simulink model "System_Modell"  (R2018a)
settings: Solver=FixedStepAuto  StartTime=0.0  StopTime=inf  FixedStep=1/f  RelTol=1e-3
values from neighbouring files (symbols this model uses):
  f = 10000    [System_Init.m]
(part 2 of 8)

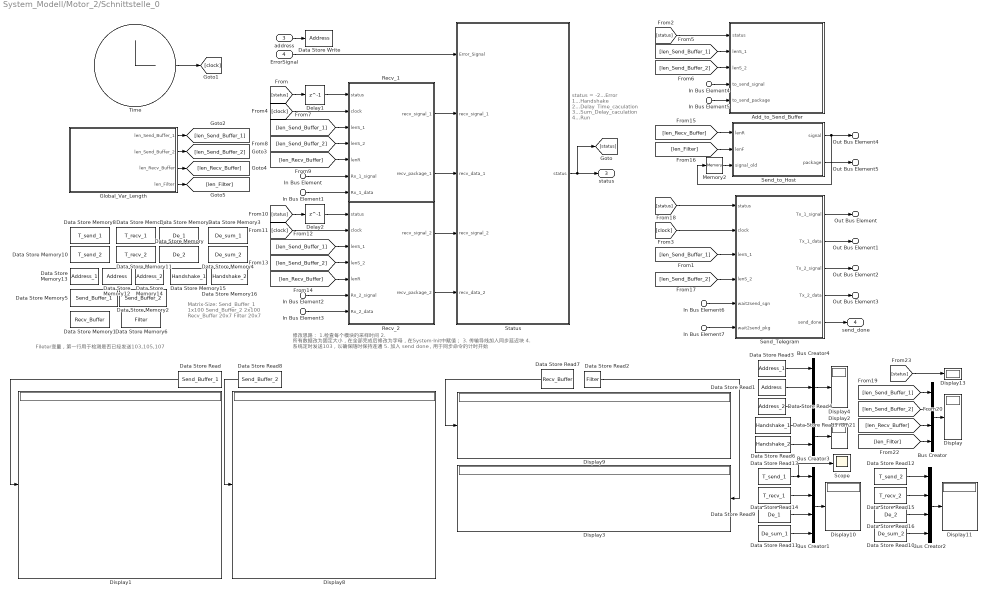
== system System_Modell/Motor_2/Schnittstelle_0 ==
  note: Fileter变量，第一行用于检测是否已经发送103,105,107
  note: 修改思路：
      | 1.检查每个模块的采样时间
      | 2. 所有数据改为固定大小，在全部完成后修改为字母，在System-Init中赋值；
      | 3. 传输导线加入同步延迟块
      | 4. 系统定时发送103，以确保随时保持连通
      | 5. 加入 send done，用于同步命令的计时开始
  note: status =
      | -2...Error
      |  1...Handshake
      |  2...Delay_Time_caculation
      |  3...Sum_Delay_caculation
      |  4...Run
  note: Matrix-Size:
      | Send_Buffer_1	1x100
      | Send_Buffer_2	2x100
      | Recv_Buffer		20x7
      | Filter			20x7
  In Bus Element : Inport  PortName=Rx_1  Element=signal
  In Bus Element1 : Inport  PortName=Rx_1  Element=data
  In Bus Element2 : Inport  Port=2  PortName=Rx_2  Element=signal
  In Bus Element3 : Inport  Port=2  PortName=Rx_2  Element=data
  address : Inport  Port=3
  ErrorSignal : Inport  Port=4
  In Bus Element4 : Inport  Port=5  PortName=wait_to_send  Element=signal
  In Bus Element6 : Inport  Port=5  PortName=wait_to_send  Element=signal
  In Bus Element5 : Inport  Port=5  PortName=wait_to_send  Element=package
  In Bus Element7 : Inport  Port=5  PortName=wait_to_send  Element=package
  Add_to_Send_Buffer : MATLAB Function  TreatAsAtomicUnit=on  SystemSampleTime=10/f
  Bus Creator : BusCreator  Inputs=4
  Bus Creator1 : BusCreator  Inputs=4
  Bus Creator2 : BusCreator  Inputs=4
  Bus Creator3 : BusCreator  Inputs=2
  Bus Creator4 : BusCreator  Inputs=3
  Data Store Memory : DataStoreMemory  DataStoreName=De_2  ReadBeforeWriteMsg=warning  WriteAfterWriteMsg=warning  WriteAfterReadMsg=warning  ShowAdditionalParam=off  OutDataTypeStr=double  Dimensions=1
  Data Store Memory1 : DataStoreMemory  DataStoreName=Recv_Buffer  ReadBeforeWriteMsg=warning  WriteAfterWriteMsg=warning  WriteAfterReadMsg=warning  InitialValue=zeros(20,7)  VectorParams1D=off  ShowAdditionalParam=off  OutDataTypeStr=double  Dimensions=[20,7]
  Data Store Memory10 : DataStoreMemory  DataStoreName=T_send_2  ReadBeforeWriteMsg=warning  WriteAfterWriteMsg=warning  WriteAfterReadMsg=warning  ShowAdditionalParam=off  OutDataTypeStr=double  Dimensions=1
  Data Store Memory11 : DataStoreMemory  DataStoreName=T_recv_2  ReadBeforeWriteMsg=warning  WriteAfterWriteMsg=warning  WriteAfterReadMsg=warning  ShowAdditionalParam=off  OutDataTypeStr=double  Dimensions=1
  Data Store Memory12 : DataStoreMemory  DataStoreName=Address  ReadBeforeWriteMsg=warning  WriteAfterWriteMsg=warning  WriteAfterReadMsg=warning  ShowAdditionalParam=off  OutDataTypeStr=double  Dimensions=1
  Data Store Memory13 : DataStoreMemory  DataStoreName=Address_1  ReadBeforeWriteMsg=warning  WriteAfterWriteMsg=warning  WriteAfterReadMsg=warning  ShowAdditionalParam=off  OutDataTypeStr=double  Dimensions=1
  Data Store Memory14 : DataStoreMemory  DataStoreName=Address_2  ReadBeforeWriteMsg=warning  WriteAfterWriteMsg=warning  WriteAfterReadMsg=warning  ShowAdditionalParam=off  OutDataTypeStr=double  Dimensions=1
  Data Store Memory15 : DataStoreMemory  DataStoreName=Handshake_1  ReadBeforeWriteMsg=warning  WriteAfterWriteMsg=warning  WriteAfterReadMsg=warning  InitialValue=false  ShowAdditionalParam=off  OutDataTypeStr=boolean
  Data Store Memory16 : DataStoreMemory  DataStoreName=Handshake_2  ReadBeforeWriteMsg=warning  WriteAfterWriteMsg=warning  WriteAfterReadMsg=warning  InitialValue=false  ShowAdditionalParam=off  OutDataTypeStr=boolean
  Data Store Memory2 : DataStoreMemory  DataStoreName=Send_Buffer_2  ReadBeforeWriteMsg=warning  WriteAfterWriteMsg=warning  WriteAfterReadMsg=warning  InitialValue=[101, 102, zeros(1,98)]  VectorParams1D=off  ShowAdditionalParam=off  OutDataTypeStr=double  Dimensions=[1,100]
  Data Store Memory3 : DataStoreMemory  DataStoreName=De_sum_1  ReadBeforeWriteMsg=warning  WriteAfterWriteMsg=warning  WriteAfterReadMsg=warning  ShowAdditionalParam=off  OutDataTypeStr=double  Dimensions=1
  Data Store Memory4 : DataStoreMemory  DataStoreName=De_sum_2  ReadBeforeWriteMsg=warning  WriteAfterWriteMsg=warning  WriteAfterReadMsg=warning  ShowAdditionalParam=off  OutDataTypeStr=double  Dimensions=1
  Data Store Memory5 : DataStoreMemory  DataStoreName=Send_Buffer_1  ReadBeforeWriteMsg=warning  WriteAfterWriteMsg=warning  WriteAfterReadMsg=warning  InitialValue=[101, 102, zeros(1,98)]  VectorParams1D=off  ShowAdditionalParam=off  OutDataTypeStr=double  Dimensions=[1,100]
  Data Store Memory6 : DataStoreMemory  DataStoreName=Filter  ReadBeforeWriteMsg=warning  WriteAfterWriteMsg=warning  WriteAfterReadMsg=warning  InitialValue=zeros(20,7)  VectorParams1D=off  ShowAdditionalParam=off  OutDataTypeStr=double  Dimensions=[20,7]
  Data Store Memory7 : DataStoreMemory  DataStoreName=De_1  ReadBeforeWriteMsg=warning  WriteAfterWriteMsg=warning  WriteAfterReadMsg=warning  ShowAdditionalParam=off  OutDataTypeStr=double  Dimensions=1
  Data Store Memory8 : DataStoreMemory  DataStoreName=T_send_1  ReadBeforeWriteMsg=warning  WriteAfterWriteMsg=warning  WriteAfterReadMsg=warning  ShowAdditionalParam=off  OutDataTypeStr=double  Dimensions=1
  Data Store Memory9 : DataStoreMemory  DataStoreName=T_recv_1  ReadBeforeWriteMsg=warning  WriteAfterWriteMsg=warning  WriteAfterReadMsg=warning  ShowAdditionalParam=off  OutDataTypeStr=double  Dimensions=1
  Data Store Read : DataStoreRead  DataStoreName=Send_Buffer_1
  Data Store Read1 : DataStoreRead  DataStoreName=Address
  Data Store Read10 : DataStoreRead  DataStoreName=De_sum_2
  Data Store Read11 : DataStoreRead  DataStoreName=De_sum_1
  Data Store Read12 : DataStoreRead  DataStoreName=T_send_2
  Data Store Read13 : DataStoreRead  DataStoreName=T_send_1
  Data Store Read14 : DataStoreRead  DataStoreName=T_recv_1
  Data Store Read15 : DataStoreRead  DataStoreName=T_recv_2
  Data Store Read16 : DataStoreRead  DataStoreName=De_2
  Data Store Read2 : DataStoreRead  DataStoreName=Filter
  Data Store Read3 : DataStoreRead  DataStoreName=Address_1
  Data Store Read4 : DataStoreRead  DataStoreName=Address_2
  Data Store Read5 : DataStoreRead  DataStoreName=Handshake_1
  Data Store Read6 : DataStoreRead  DataStoreName=Handshake_2
  Data Store Read7 : DataStoreRead  DataStoreName=Recv_Buffer
  Data Store Read8 : DataStoreRead  DataStoreName=Send_Buffer_2
  Data Store Read9 : DataStoreRead  DataStoreName=De_1
  Data Store Write : DataStoreWrite  DataStoreName=Address
  Delay1 : Delay  DelayLength=1
  Delay2 : Delay  DelayLength=1
  Display{,1..4,8..11,13} (10 alike) : Display
  Global_Var_Length : MATLAB Function  TreatAsAtomicUnit=on
  Memory2 : Memory  InitialCondition=false
  Recv_1 : MATLAB Function  TreatAsAtomicUnit=on  SystemSampleTime=10/f
  Recv_2 : MATLAB Function  TreatAsAtomicUnit=on  SystemSampleTime=10/f
  Scope : Scope
  Send_Telegram : Subsystem
  Send_to_Host : MATLAB Function  TreatAsAtomicUnit=on  SystemSampleTime=10/f
  Status : Stateflow chart  TreatAsAtomicUnit=on
  Time : Clock
      settings: Decimation=f
  Out Bus Element : Outport  PortName=Tx_1  Element=signal
  Out Bus Element1 : Outport  PortName=Tx_1  Element=data
  Out Bus Element2 : Outport  Port=2  PortName=Tx_2  Element=signal
  Out Bus Element3 : Outport  Port=2  PortName=Tx_2  Element=data
  status : Outport  Port=3
  send_done : Outport  Port=4
  Out Bus Element4 : Outport  Port=5  PortName=Recv  Element=signal
  Out Bus Element5 : Outport  Port=5  PortName=Recv  Element=package
  wires:
  ErrorSignal/1 -> Status/1(Error_Signal)
  Status/1(status) -> [status], status/1
  In Bus Element1/1 -> Recv_1/7(Rx_1_data)
  In Bus Element/1 -> Recv_1/6(Rx_1_signal)
  [status] -> Delay1/1
  Time/1 -> [clock]
  [clock] -> Recv_1/2(clock)
  Send_to_Host/1(signal) -> Out Bus Element4/1, Memory2/1
  address/1 -> Data Store Write/1
  Global_Var_Length/1(len_Send_Buffer_1) -> [len_Send_Buffer_1]
  Global_Var_Length/2(len_Send_Buffer_2) -> [len_Send_Buffer_2]
  Global_Var_Length/3(len_Recv_Buffer) -> [len_Recv_Buffer]
  Global_Var_Length/4(len_Filter) -> [len_Filter]
  [len_Send_Buffer_1] -> Recv_1/3(lenS_1)
  [len_Send_Buffer_2] -> Recv_1/4(lenS_2)
  [len_Recv_Buffer] -> Recv_1/5(lenR)
  In Bus Element2/1 -> Recv_2/6(Rx_2_signal)
  In Bus Element3/1 -> Recv_2/7(Rx_2_data)
  [status] -> Delay2/1
  [len_Recv_Buffer] -> Recv_2/5(lenR)
  [len_Send_Buffer_1] -> Recv_2/3(lenS_1)
  [clock] -> Recv_2/2(clock)
  [len_Send_Buffer_2] -> Recv_2/4(lenS_2)
  Delay1/1 -> Recv_1/1(status)
  Delay2/1 -> Recv_2/1(status)
  Recv_1/1(recv_signal_1) -> Status/2(recv_signal_1)
  Recv_1/2(recv_package_1) -> Status/3(recv_data_1)
  Recv_2/1(recv_signal_2) -> Status/4(recv_signal_2)
  Recv_2/2(recv_package_2) -> Status/5(recv_data_2)
  [len_Recv_Buffer] -> Send_to_Host/1(lenR)
  [len_Filter] -> Send_to_Host/2(lenF)
  [len_Send_Buffer_1] -> Add_to_Send_Buffer/2(lenS_1)
  [len_Send_Buffer_2] -> Add_to_Send_Buffer/3(lenS_2)
  In Bus Element4/1 -> Add_to_Send_Buffer/4(to_send_signal)
  In Bus Element5/1 -> Add_to_Send_Buffer/5(to_send_package)
  [status] -> Add_to_Send_Buffer/1(status)
  Memory2/1 -> Send_to_Host/3(signal_old)
  Bus Creator/1 -> Display/1
  [len_Send_Buffer_1] -> Bus Creator/1
  [len_Send_Buffer_2] -> Bus Creator/2
  [len_Recv_Buffer] -> Bus Creator/3
  [len_Filter] -> Bus Creator/4
  Data Store Read/1 -> Display1/1
  Data Store Read2/1 -> Display3/1
  Data Store Read8/1 -> Display8/1
  Data Store Read7/1 -> Display9/1
  Data Store Read13/1 -> Scope/1, Bus Creator1/1
  Data Store Read14/1 -> Bus Creator1/2
  Data Store Read11/1 -> Bus Creator1/4
  Data Store Read9/1 -> Bus Creator1/3
  Bus Creator1/1 -> Display10/1
  Data Store Read12/1 -> Bus Creator2/1
  Data Store Read15/1 -> Bus Creator2/2
  Bus Creator2/1 -> Display11/1
  Data Store Read16/1 -> Bus Creator2/3
  Data Store Read10/1 -> Bus Creator2/4
  [status] -> Display13/1
  Send_to_Host/2(package) -> Out Bus Element5/1
  Data Store Read5/1 -> Bus Creator3/1
  Data Store Read6/1 -> Bus Creator3/2
  Data Store Read4/1 -> Bus Creator4/3
  Data Store Read1/1 -> Bus Creator4/2
  Data Store Read3/1 -> Bus Creator4/1
  Bus Creator3/1 -> Display2/1
  Bus Creator4/1 -> Display4/1
  [status] -> Send_Telegram/1(status)
  [clock] -> Send_Telegram/2(clock)
  [len_Send_Buffer_1] -> Send_Telegram/3(lenS_1)
  [len_Send_Buffer_2] -> Send_Telegram/4(lenS_2)
  Send_Telegram/3(Tx_2_signal) -> Out Bus Element2/1
  Send_Telegram/4(Tx_2_data) -> Out Bus Element3/1
  Send_Telegram/2(Tx_1_data) -> Out Bus Element1/1
  Send_Telegram/1(Tx_1_signal) -> Out Bus Element/1
  Send_Telegram/5(send_done) -> send_done/1
  In Bus Element6/1 -> Send_Telegram/5(wait2send_sgn)
  In Bus Element7/1 -> Send_Telegram/6(wait2send_pkg)

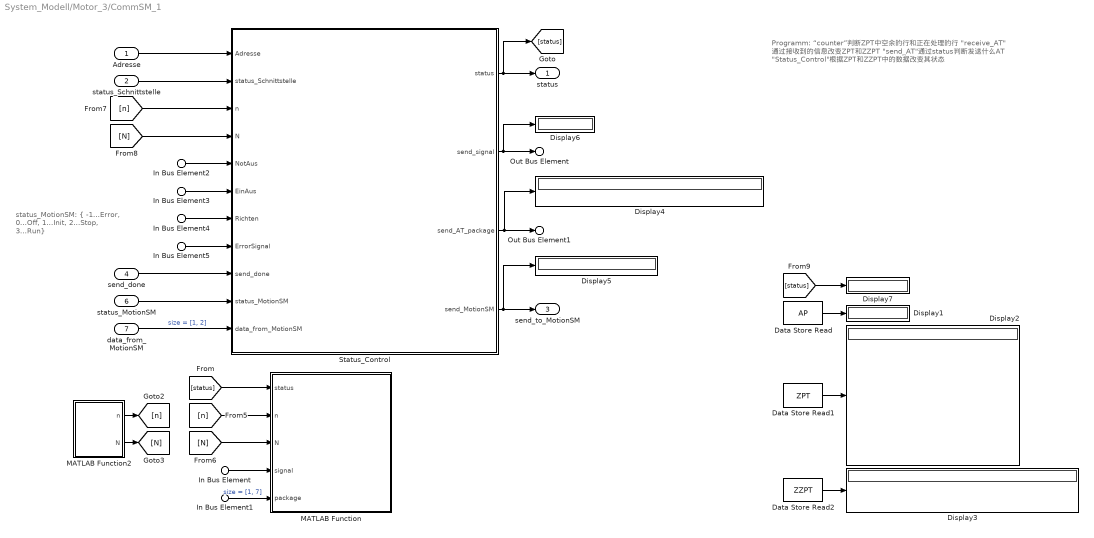
== system System_Modell/Motor_3/CommSM_1 ==
  note: Programm:
      | “counter”判断ZPT中空余的行和正在处理的行
      | "receive_AT" 通过接收到的信息改变ZPT和ZZPT
      | "send_AT"通过status判断发送什么AT
      | "Status_Control"根据ZPT和ZZPT中的数据改变其状态
  note: status_MotionSM: {
      | -1...Error,
      | 0...Off,
      | 1...Init,
      | 2...Stop,
      | 3...Run}
  Adresse : Inport  OutDataTypeStr=double  PortDimensions=1
  status_Schnittstelle : Inport  Port=2  OutDataTypeStr=double  PortDimensions=1
  In Bus Element2 : Inport  Port=3  PortName=Control  Element=NotAus
  In Bus Element3 : Inport  Port=3  PortName=Control  Element=EinAus
  In Bus Element4 : Inport  Port=3  PortName=Control  Element=Richten
  In Bus Element5 : Inport  Port=3  PortName=Control  Element=ErrorSignal
  send_done : Inport  Port=4
  In Bus Element : Inport  Port=5  PortName=Recv  Element=signal
  In Bus Element1 : Inport  Port=5  PortName=Recv  Element=package
  status_MotionSM : Inport  Port=6  OutDataTypeStr=double  PortDimensions=1
  data_from_MotionSM : Inport  Port=7  OutDataTypeStr=double  PortDimensions=2
  Data Store Read : DataStoreRead  DataStoreName=AP
  Data Store Read1 : DataStoreRead  DataStoreName=ZPT
  Data Store Read2 : DataStoreRead  DataStoreName=ZZPT
  Display{1..7} (7 alike) : Display
  MATLAB Function : MATLAB Function  TreatAsAtomicUnit=on
  MATLAB Function2 : MATLAB Function  TreatAsAtomicUnit=on
  Status_Control : Stateflow chart  TreatAsAtomicUnit=on
  status : Outport  OutDataTypeStr=double  PortDimensions=1
  Out Bus Element : Outport  Port=2  PortName=data_to_send  Element=signal
  Out Bus Element1 : Outport  Port=2  PortName=data_to_send  Element=package
  send_to_MotionSM : Outport  Port=3
  wires:
  In Bus Element2/1 -> Status_Control/5(NotAus)
  In Bus Element3/1 -> Status_Control/6(EinAus)
  In Bus Element4/1 -> Status_Control/7(Richten)
  In Bus Element5/1 -> Status_Control/8(ErrorSignal)
  status_Schnittstelle/1 -> Status_Control/2(status_Schnittstelle)
  In Bus Element/1 -> MATLAB Function/4(signal)
  In Bus Element1/1 -> MATLAB Function/5(package)  "size = [1, 7]"
  data_from_MotionSM/1 -> Status_Control/11(data_from_MotionSM)  "size = [1, 2]"
  status_MotionSM/1 -> Status_Control/10(status_MotionSM)
  Adresse/1 -> Status_Control/1(Adresse)
  Status_Control/1(status) -> [status], status/1
  Status_Control/3(send_AT_package) -> Out Bus Element1/1, Display4/1
  Status_Control/4(send_MotionSM) -> send_to_MotionSM/1, Display5/1
  Status_Control/2(send_signal) -> Out Bus Element/1, Display6/1
  Data Store Read/1 -> Display1/1
  Data Store Read1/1 -> Display2/1
  Data Store Read2/1 -> Display3/1
  [status] -> MATLAB Function/1(status)
  MATLAB Function2/1(n) -> [n]
  MATLAB Function2/2(N) -> [N]
  [N] -> MATLAB Function/3(N)
  [n] -> MATLAB Function/2(n)
  [n] -> Status_Control/3(n)
  [N] -> Status_Control/4(N)
  [status] -> Display7/1
  send_done/1 -> Status_Control/9(send_done)

== system System_Modell/Motor_3/MotionSM_1 ==
  note: parameter = [delta_T, a_max, v_max, s0]
  In Bus Element : Inport  PortName=Control  Element=NotAus
  In Bus Element1 : Inport  PortName=Control  Element=EinAus
  In Bus Element2 : Inport  PortName=Control  Element=Richten
  In Bus Element3 : Inport  PortName=Control  Element=ErrorSignal
  data_received : Inport  Port=2  OutDataTypeStr=double  PortDimensions=2
  delta_T : Inport  Port=3
  Bus Creator : BusCreator  Inputs=3
  Chart : Stateflow chart  TreatAsAtomicUnit=on
  Data Store Read : DataStoreRead  DataStoreName=AP
  Delay : Delay  DelayLength=1
  Delay1 : Delay  DelayLength=1
  Display{1..2,4..7} (6 alike) : Display
  MATLAB Function : MATLAB Function  TreatAsAtomicUnit=on
  Motor : Subsystem
  status : Outport
  data_to_send : Outport  Port=2  OutDataTypeStr=double  PortDimensions=2
  Out Bus Element : Outport  Port=3  PortName=Par  Element=a
  Out Bus Element1 : Outport  Port=3  PortName=Par  Element=v
  Out Bus Element2 : Outport  Port=3  PortName=Par  Element=s
  Out Bus Element3 : Outport  Port=3  PortName=Par  Element=AP
  wires:
  Chart/1(status) -> Motor/1(auto_control), Delay/1, Display1/1, status/1
  In Bus Element1/1 -> Chart/2(EinAus)
  In Bus Element/1 -> Chart/1(NotAus)
  In Bus Element2/1 -> Chart/3(Richten)
  In Bus Element3/1 -> Chart/4(ErrorSignal)
  Motor/1(status_Motor) -> Display4/1, Delay1/1
  data_received/1 -> MATLAB Function/2(data_received)
  Delay1/1 -> Chart/6(Motor_status)
  MATLAB Function/1(excute_signal) -> Display6/1, Chart/5(excute_signal)
  MATLAB Function/2(message_to_send) -> data_to_send/1, Display7/1  "size = [1, 2]"
  delta_T/1 -> Chart/7(delta_T)
  Motor/2(a) -> Bus Creator/3, Out Bus Element/1
  Motor/3(v) -> Bus Creator/2, Out Bus Element1/1
  Motor/4(s) -> Bus Creator/1, Out Bus Element2/1
  Chart/2(parameter) -> Motor/2(parameter), Display5/1
  Delay/1 -> MATLAB Function/1(status)
  Data Store Read/1 -> Out Bus Element3/1
  Bus Creator/1 -> Display2/1

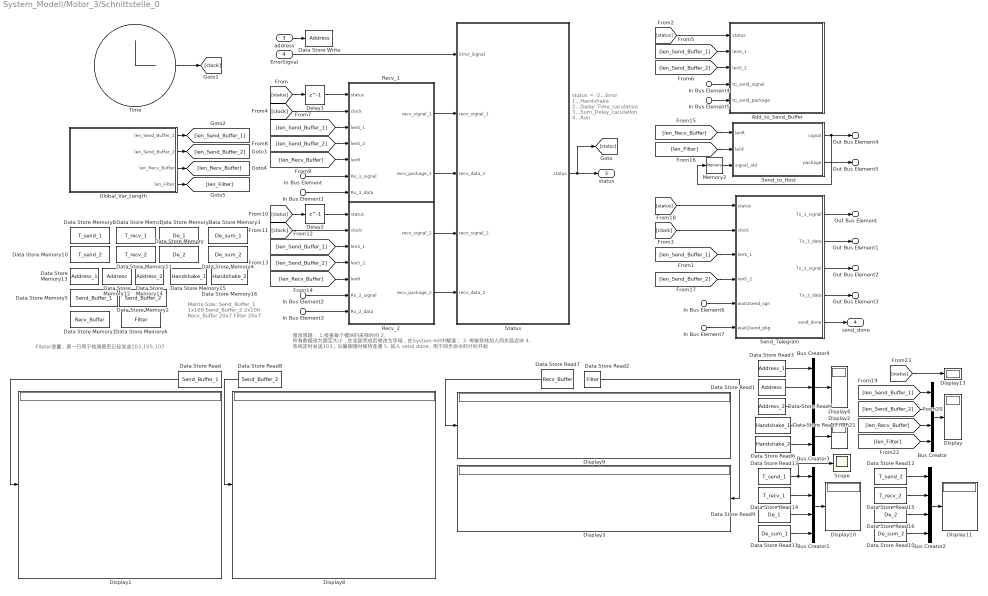
== system System_Modell/Motor_3/Schnittstelle_0 ==
  note: Fileter变量，第一行用于检测是否已经发送103,105,107
  note: 修改思路：
      | 1.检查每个模块的采样时间
      | 2. 所有数据改为固定大小，在全部完成后修改为字母，在System-Init中赋值；
      | 3. 传输导线加入同步延迟块
      | 4. 系统定时发送103，以确保随时保持连通
      | 5. 加入 send done，用于同步命令的计时开始
  note: status =
      | -2...Error
      |  1...Handshake
      |  2...Delay_Time_caculation
      |  3...Sum_Delay_caculation
      |  4...Run
  note: Matrix-Size:
      | Send_Buffer_1	1x100
      | Send_Buffer_2	2x100
      | Recv_Buffer		20x7
      | Filter			20x7
  In Bus Element : Inport  PortName=Rx_1  Element=signal
  In Bus Element1 : Inport  PortName=Rx_1  Element=data
  In Bus Element2 : Inport  Port=2  PortName=Rx_2  Element=signal
  In Bus Element3 : Inport  Port=2  PortName=Rx_2  Element=data
  address : Inport  Port=3
  ErrorSignal : Inport  Port=4
  In Bus Element4 : Inport  Port=5  PortName=wait_to_send  Element=signal
  In Bus Element6 : Inport  Port=5  PortName=wait_to_send  Element=signal
  In Bus Element5 : Inport  Port=5  PortName=wait_to_send  Element=package
  In Bus Element7 : Inport  Port=5  PortName=wait_to_send  Element=package
  Add_to_Send_Buffer : MATLAB Function  TreatAsAtomicUnit=on  SystemSampleTime=10/f
  Bus Creator : BusCreator  Inputs=4
  Bus Creator1 : BusCreator  Inputs=4
  Bus Creator2 : BusCreator  Inputs=4
  Bus Creator3 : BusCreator  Inputs=2
  Bus Creator4 : BusCreator  Inputs=3
  Data Store Memory : DataStoreMemory  DataStoreName=De_2  ReadBeforeWriteMsg=warning  WriteAfterWriteMsg=warning  WriteAfterReadMsg=warning  ShowAdditionalParam=off  OutDataTypeStr=double  Dimensions=1
  Data Store Memory1 : DataStoreMemory  DataStoreName=Recv_Buffer  ReadBeforeWriteMsg=warning  WriteAfterWriteMsg=warning  WriteAfterReadMsg=warning  InitialValue=zeros(20,7)  VectorParams1D=off  ShowAdditionalParam=off  OutDataTypeStr=double  Dimensions=[20,7]
  Data Store Memory10 : DataStoreMemory  DataStoreName=T_send_2  ReadBeforeWriteMsg=warning  WriteAfterWriteMsg=warning  WriteAfterReadMsg=warning  ShowAdditionalParam=off  OutDataTypeStr=double  Dimensions=1
  Data Store Memory11 : DataStoreMemory  DataStoreName=T_recv_2  ReadBeforeWriteMsg=warning  WriteAfterWriteMsg=warning  WriteAfterReadMsg=warning  ShowAdditionalParam=off  OutDataTypeStr=double  Dimensions=1
  Data Store Memory12 : DataStoreMemory  DataStoreName=Address  ReadBeforeWriteMsg=warning  WriteAfterWriteMsg=warning  WriteAfterReadMsg=warning  ShowAdditionalParam=off  OutDataTypeStr=double  Dimensions=1
  Data Store Memory13 : DataStoreMemory  DataStoreName=Address_1  ReadBeforeWriteMsg=warning  WriteAfterWriteMsg=warning  WriteAfterReadMsg=warning  ShowAdditionalParam=off  OutDataTypeStr=double  Dimensions=1
  Data Store Memory14 : DataStoreMemory  DataStoreName=Address_2  ReadBeforeWriteMsg=warning  WriteAfterWriteMsg=warning  WriteAfterReadMsg=warning  ShowAdditionalParam=off  OutDataTypeStr=double  Dimensions=1
  Data Store Memory15 : DataStoreMemory  DataStoreName=Handshake_1  ReadBeforeWriteMsg=warning  WriteAfterWriteMsg=warning  WriteAfterReadMsg=warning  InitialValue=false  ShowAdditionalParam=off  OutDataTypeStr=boolean
  Data Store Memory16 : DataStoreMemory  DataStoreName=Handshake_2  ReadBeforeWriteMsg=warning  WriteAfterWriteMsg=warning  WriteAfterReadMsg=warning  InitialValue=false  ShowAdditionalParam=off  OutDataTypeStr=boolean
  Data Store Memory2 : DataStoreMemory  DataStoreName=Send_Buffer_2  ReadBeforeWriteMsg=warning  WriteAfterWriteMsg=warning  WriteAfterReadMsg=warning  InitialValue=[101, 102, zeros(1,98)]  VectorParams1D=off  ShowAdditionalParam=off  OutDataTypeStr=double  Dimensions=[1,100]
  Data Store Memory3 : DataStoreMemory  DataStoreName=De_sum_1  ReadBeforeWriteMsg=warning  WriteAfterWriteMsg=warning  WriteAfterReadMsg=warning  ShowAdditionalParam=off  OutDataTypeStr=double  Dimensions=1
  Data Store Memory4 : DataStoreMemory  DataStoreName=De_sum_2  ReadBeforeWriteMsg=warning  WriteAfterWriteMsg=warning  WriteAfterReadMsg=warning  ShowAdditionalParam=off  OutDataTypeStr=double  Dimensions=1
  Data Store Memory5 : DataStoreMemory  DataStoreName=Send_Buffer_1  ReadBeforeWriteMsg=warning  WriteAfterWriteMsg=warning  WriteAfterReadMsg=warning  InitialValue=[101, 102, zeros(1,98)]  VectorParams1D=off  ShowAdditionalParam=off  OutDataTypeStr=double  Dimensions=[1,100]
  Data Store Memory6 : DataStoreMemory  DataStoreName=Filter  ReadBeforeWriteMsg=warning  WriteAfterWriteMsg=warning  WriteAfterReadMsg=warning  InitialValue=zeros(20,7)  VectorParams1D=off  ShowAdditionalParam=off  OutDataTypeStr=double  Dimensions=[20,7]
  Data Store Memory7 : DataStoreMemory  DataStoreName=De_1  ReadBeforeWriteMsg=warning  WriteAfterWriteMsg=warning  WriteAfterReadMsg=warning  ShowAdditionalParam=off  OutDataTypeStr=double  Dimensions=1
  Data Store Memory8 : DataStoreMemory  DataStoreName=T_send_1  ReadBeforeWriteMsg=warning  WriteAfterWriteMsg=warning  WriteAfterReadMsg=warning  ShowAdditionalParam=off  OutDataTypeStr=double  Dimensions=1
  Data Store Memory9 : DataStoreMemory  DataStoreName=T_recv_1  ReadBeforeWriteMsg=warning  WriteAfterWriteMsg=warning  WriteAfterReadMsg=warning  ShowAdditionalParam=off  OutDataTypeStr=double  Dimensions=1
  Data Store Read : DataStoreRead  DataStoreName=Send_Buffer_1
  Data Store Read1 : DataStoreRead  DataStoreName=Address
  Data Store Read10 : DataStoreRead  DataStoreName=De_sum_2
  Data Store Read11 : DataStoreRead  DataStoreName=De_sum_1
  Data Store Read12 : DataStoreRead  DataStoreName=T_send_2
  Data Store Read13 : DataStoreRead  DataStoreName=T_send_1
  Data Store Read14 : DataStoreRead  DataStoreName=T_recv_1
  Data Store Read15 : DataStoreRead  DataStoreName=T_recv_2
  Data Store Read16 : DataStoreRead  DataStoreName=De_2
  Data Store Read2 : DataStoreRead  DataStoreName=Filter
  Data Store Read3 : DataStoreRead  DataStoreName=Address_1
  Data Store Read4 : DataStoreRead  DataStoreName=Address_2
  Data Store Read5 : DataStoreRead  DataStoreName=Handshake_1
  Data Store Read6 : DataStoreRead  DataStoreName=Handshake_2
  Data Store Read7 : DataStoreRead  DataStoreName=Recv_Buffer
  Data Store Read8 : DataStoreRead  DataStoreName=Send_Buffer_2
  Data Store Read9 : DataStoreRead  DataStoreName=De_1
  Data Store Write : DataStoreWrite  DataStoreName=Address
  Delay1 : Delay  DelayLength=1
  Delay2 : Delay  DelayLength=1
  Display{,1..4,8..11,13} (10 alike) : Display
  Global_Var_Length : MATLAB Function  TreatAsAtomicUnit=on
  Memory2 : Memory  InitialCondition=false
  Recv_1 : MATLAB Function  TreatAsAtomicUnit=on  SystemSampleTime=10/f
  Recv_2 : MATLAB Function  TreatAsAtomicUnit=on  SystemSampleTime=10/f
  Scope : Scope
  Send_Telegram : Subsystem
  Send_to_Host : MATLAB Function  TreatAsAtomicUnit=on  SystemSampleTime=10/f
  Status : Stateflow chart  TreatAsAtomicUnit=on
  Time : Clock
      settings: Decimation=f
  Out Bus Element : Outport  PortName=Tx_1  Element=signal
  Out Bus Element1 : Outport  PortName=Tx_1  Element=data
  Out Bus Element2 : Outport  Port=2  PortName=Tx_2  Element=signal
  Out Bus Element3 : Outport  Port=2  PortName=Tx_2  Element=data
  status : Outport  Port=3
  send_done : Outport  Port=4
  Out Bus Element4 : Outport  Port=5  PortName=Recv  Element=signal
  Out Bus Element5 : Outport  Port=5  PortName=Recv  Element=package
  wires:
  ErrorSignal/1 -> Status/1(Error_Signal)
  Status/1(status) -> [status], status/1
  In Bus Element1/1 -> Recv_1/7(Rx_1_data)
  In Bus Element/1 -> Recv_1/6(Rx_1_signal)
  [status] -> Delay1/1
  Time/1 -> [clock]
  [clock] -> Recv_1/2(clock)
  Send_to_Host/1(signal) -> Out Bus Element4/1, Memory2/1
  address/1 -> Data Store Write/1
  Global_Var_Length/1(len_Send_Buffer_1) -> [len_Send_Buffer_1]
  Global_Var_Length/2(len_Send_Buffer_2) -> [len_Send_Buffer_2]
  Global_Var_Length/3(len_Recv_Buffer) -> [len_Recv_Buffer]
  Global_Var_Length/4(len_Filter) -> [len_Filter]
  [len_Send_Buffer_1] -> Recv_1/3(lenS_1)
  [len_Send_Buffer_2] -> Recv_1/4(lenS_2)
  [len_Recv_Buffer] -> Recv_1/5(lenR)
  In Bus Element2/1 -> Recv_2/6(Rx_2_signal)
  In Bus Element3/1 -> Recv_2/7(Rx_2_data)
  [status] -> Delay2/1
  [len_Recv_Buffer] -> Recv_2/5(lenR)
  [len_Send_Buffer_1] -> Recv_2/3(lenS_1)
  [clock] -> Recv_2/2(clock)
  [len_Send_Buffer_2] -> Recv_2/4(lenS_2)
  Delay1/1 -> Recv_1/1(status)
  Delay2/1 -> Recv_2/1(status)
  Recv_1/1(recv_signal_1) -> Status/2(recv_signal_1)
  Recv_1/2(recv_package_1) -> Status/3(recv_data_1)
  Recv_2/1(recv_signal_2) -> Status/4(recv_signal_2)
  Recv_2/2(recv_package_2) -> Status/5(recv_data_2)
  [len_Recv_Buffer] -> Send_to_Host/1(lenR)
  [len_Filter] -> Send_to_Host/2(lenF)
  [len_Send_Buffer_1] -> Add_to_Send_Buffer/2(lenS_1)
  [len_Send_Buffer_2] -> Add_to_Send_Buffer/3(lenS_2)
  In Bus Element4/1 -> Add_to_Send_Buffer/4(to_send_signal)
  In Bus Element5/1 -> Add_to_Send_Buffer/5(to_send_package)
  [status] -> Add_to_Send_Buffer/1(status)
  Memory2/1 -> Send_to_Host/3(signal_old)
  Bus Creator/1 -> Display/1
  [len_Send_Buffer_1] -> Bus Creator/1
  [len_Send_Buffer_2] -> Bus Creator/2
  [len_Recv_Buffer] -> Bus Creator/3
  [len_Filter] -> Bus Creator/4
  Data Store Read/1 -> Display1/1
  Data Store Read2/1 -> Display3/1
  Data Store Read8/1 -> Display8/1
  Data Store Read7/1 -> Display9/1
  Data Store Read13/1 -> Scope/1, Bus Creator1/1
  Data Store Read14/1 -> Bus Creator1/2
  Data Store Read11/1 -> Bus Creator1/4
  Data Store Read9/1 -> Bus Creator1/3
  Bus Creator1/1 -> Display10/1
  Data Store Read12/1 -> Bus Creator2/1
  Data Store Read15/1 -> Bus Creator2/2
  Bus Creator2/1 -> Display11/1
  Data Store Read16/1 -> Bus Creator2/3
  Data Store Read10/1 -> Bus Creator2/4
  [status] -> Display13/1
  Send_to_Host/2(package) -> Out Bus Element5/1
  Data Store Read5/1 -> Bus Creator3/1
  Data Store Read6/1 -> Bus Creator3/2
  Data Store Read4/1 -> Bus Creator4/3
  Data Store Read1/1 -> Bus Creator4/2
  Data Store Read3/1 -> Bus Creator4/1
  Bus Creator3/1 -> Display2/1
  Bus Creator4/1 -> Display4/1
  [status] -> Send_Telegram/1(status)
  [clock] -> Send_Telegram/2(clock)
  [len_Send_Buffer_1] -> Send_Telegram/3(lenS_1)
  [len_Send_Buffer_2] -> Send_Telegram/4(lenS_2)
  Send_Telegram/3(Tx_2_signal) -> Out Bus Element2/1
  Send_Telegram/4(Tx_2_data) -> Out Bus Element3/1
  Send_Telegram/2(Tx_1_data) -> Out Bus Element1/1
  Send_Telegram/1(Tx_1_signal) -> Out Bus Element/1
  Send_Telegram/5(send_done) -> send_done/1
  In Bus Element6/1 -> Send_Telegram/5(wait2send_sgn)
  In Bus Element7/1 -> Send_Telegram/6(wait2send_pkg)

== system System_Modell/ZP_Mananger/GSM  ==
  note: package= [n, Ax1, status, n, Ax2, status, n, Ax3, status]
  note: Update_data = [sender, receiver, cmd=113, n, Ax, status, delay]
  In Bus Element6 : Inport  PortName=Recv  Element=signal
  In Bus Element7 : Inport  PortName=Recv  Element=package
  Schnittstelle_status : Inport  Port=2  OutDataTypeStr=double
  In Bus Element4 : Inport  Port=3  PortName=SkillRequest  Element=signal
  In Bus Element5 : Inport  Port=3  PortName=SkillRequest  Element=request
  Adresse : Inport  Port=4
  In Bus Element : Inport  Port=5  PortName=Control  Element=NotAus
  In Bus Element1 : Inport  Port=5  PortName=Control  Element=EinAus
  In Bus Element2 : Inport  Port=5  PortName=Control  Element=Richten
  In Bus Element3 : Inport  Port=5  PortName=Control  Element=ErrorSignal
  Delay : Delay  DelayLength=1
  Delay1 : Delay  DelayLength=1
  Display{1..4,7} (5 alike) : Display
  State Machine : Stateflow chart  TreatAsAtomicUnit=on
  ZP-Tabelle bearbeiten : Subsystem
  Out Bus Element : Outport  PortName=data_to_send  Element=signal
  Out Bus Element1 : Outport  PortName=data_to_send  Element=package
  status : Outport  Port=2
  wires:
  In Bus Element6/1 -> State Machine/8(received_signal)
  In Bus Element2/1 -> State Machine/3(Richten)
  State Machine/1(status) -> Display7/1, [status], status/1
  In Bus Element/1 -> State Machine/1(NotAus)
  In Bus Element1/1 -> State Machine/2(EinAus)
  Schnittstelle_status/1 -> State Machine/7(Schnittstelle_status)
  State Machine/4(GSM_ErrorCode) -> Display1/1
  In Bus Element4/1 -> State Machine/5(SkillRequest_signal), ZP-Tabelle bearbeiten/2(SkillRequest_signal)
  In Bus Element5/1 -> ZP-Tabelle bearbeiten/4(SkillRequest)
  In Bus Element3/1 -> State Machine/4(GSM_Error)
  State Machine/2(send_signal) -> Out Bus Element/1
  State Machine/3(Data_Package) -> Out Bus Element1/1, Display2/1
  In Bus Element7/1 -> ZP-Tabelle bearbeiten/6(Update_data)
  ZP-Tabelle bearbeiten/1(send_SkillRequest) -> State Machine/6(SkillRequest_package), Display4/1
  ZP-Tabelle bearbeiten/2(Update_done) -> Display3/1, State Machine/9(update_done)
  State Machine/5(Update_signal) -> Delay/1
  Delay/1 -> ZP-Tabelle bearbeiten/5(Update_signal)
  Adresse/1 -> ZP-Tabelle bearbeiten/3(Adresse)
  [status] -> Delay1/1
  Delay1/1 -> ZP-Tabelle bearbeiten/1(status)

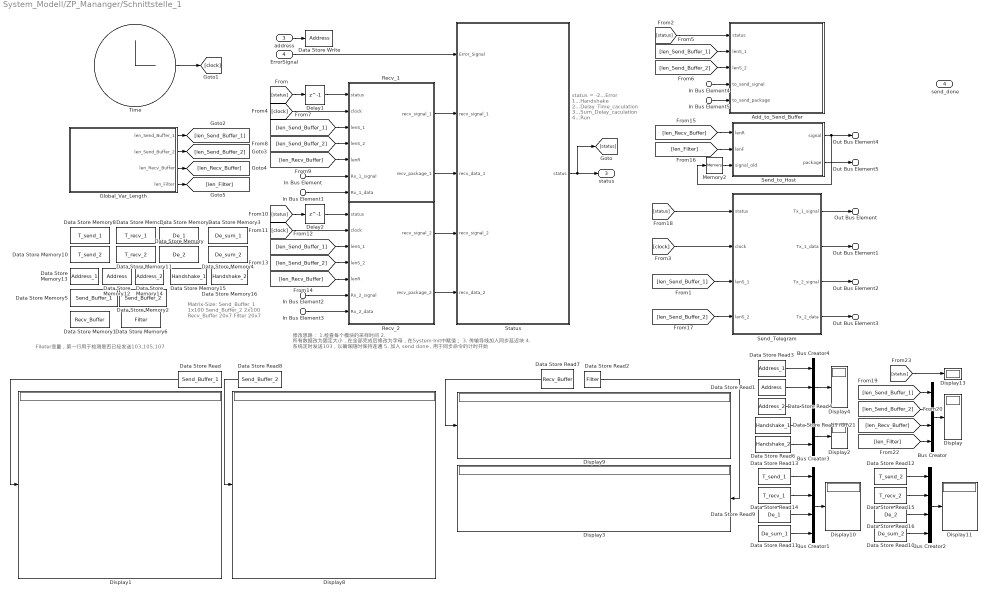
== system System_Modell/ZP_Mananger/Schnittstelle_1 ==
  note: Fileter变量，第一行用于检测是否已经发送103,105,107
  note: 修改思路：
      | 1.检查每个模块的采样时间
      | 2. 所有数据改为固定大小，在全部完成后修改为字母，在System-Init中赋值；
      | 3. 传输导线加入同步延迟块
      | 4. 系统定时发送103，以确保随时保持连通
      | 5. 加入 send done，用于同步命令的计时开始
  note: status =
      | -2...Error
      |  1...Handshake
      |  2...Delay_Time_caculation
      |  3...Sum_Delay_caculation
      |  4...Run
  note: Matrix-Size:
      | Send_Buffer_1	1x100
      | Send_Buffer_2	2x100
      | Recv_Buffer		20x7
      | Filter			20x7
  In Bus Element : Inport  PortName=Rx_1  Element=signal
  In Bus Element1 : Inport  PortName=Rx_1  Element=data
  In Bus Element2 : Inport  Port=2  PortName=Rx_2  Element=signal
  In Bus Element3 : Inport  Port=2  PortName=Rx_2  Element=data
  address : Inport  Port=3
  ErrorSignal : Inport  Port=4
  In Bus Element4 : Inport  Port=5  PortName=wait_to_send  Element=signal
  In Bus Element5 : Inport  Port=5  PortName=wait_to_send  Element=package
  Add_to_Send_Buffer : MATLAB Function  TreatAsAtomicUnit=on  SystemSampleTime=10/f
  Bus Creator : BusCreator  Inputs=4
  Bus Creator1 : BusCreator  Inputs=4
  Bus Creator2 : BusCreator  Inputs=4
  Bus Creator3 : BusCreator  Inputs=2
  Bus Creator4 : BusCreator  Inputs=3
  Data Store Memory : DataStoreMemory  DataStoreName=De_2  ReadBeforeWriteMsg=warning  WriteAfterWriteMsg=warning  WriteAfterReadMsg=warning  ShowAdditionalParam=off  OutDataTypeStr=double  Dimensions=1
  Data Store Memory1 : DataStoreMemory  DataStoreName=Recv_Buffer  ReadBeforeWriteMsg=warning  WriteAfterWriteMsg=warning  WriteAfterReadMsg=warning  InitialValue=zeros(20,7)  VectorParams1D=off  ShowAdditionalParam=off  OutDataTypeStr=double  Dimensions=[20,7]
  Data Store Memory10 : DataStoreMemory  DataStoreName=T_send_2  ReadBeforeWriteMsg=warning  WriteAfterWriteMsg=warning  WriteAfterReadMsg=warning  ShowAdditionalParam=off  OutDataTypeStr=double  Dimensions=1
  Data Store Memory11 : DataStoreMemory  DataStoreName=T_recv_2  ReadBeforeWriteMsg=warning  WriteAfterWriteMsg=warning  WriteAfterReadMsg=warning  ShowAdditionalParam=off  OutDataTypeStr=double  Dimensions=1
  Data Store Memory12 : DataStoreMemory  DataStoreName=Address  ReadBeforeWriteMsg=warning  WriteAfterWriteMsg=warning  WriteAfterReadMsg=warning  ShowAdditionalParam=off  OutDataTypeStr=double  Dimensions=1
  Data Store Memory13 : DataStoreMemory  DataStoreName=Address_1  ReadBeforeWriteMsg=warning  WriteAfterWriteMsg=warning  WriteAfterReadMsg=warning  ShowAdditionalParam=off  OutDataTypeStr=double  Dimensions=1
  Data Store Memory14 : DataStoreMemory  DataStoreName=Address_2  ReadBeforeWriteMsg=warning  WriteAfterWriteMsg=warning  WriteAfterReadMsg=warning  ShowAdditionalParam=off  OutDataTypeStr=double  Dimensions=1
  Data Store Memory15 : DataStoreMemory  DataStoreName=Handshake_1  ReadBeforeWriteMsg=warning  WriteAfterWriteMsg=warning  WriteAfterReadMsg=warning  InitialValue=false  ShowAdditionalParam=off  OutDataTypeStr=boolean
  Data Store Memory16 : DataStoreMemory  DataStoreName=Handshake_2  ReadBeforeWriteMsg=warning  WriteAfterWriteMsg=warning  WriteAfterReadMsg=warning  InitialValue=false  ShowAdditionalParam=off  OutDataTypeStr=boolean
  Data Store Memory2 : DataStoreMemory  DataStoreName=Send_Buffer_2  ReadBeforeWriteMsg=warning  WriteAfterWriteMsg=warning  WriteAfterReadMsg=warning  InitialValue=[101, 102, zeros(1,98)]  VectorParams1D=off  ShowAdditionalParam=off  OutDataTypeStr=double  Dimensions=[1,100]
  Data Store Memory3 : DataStoreMemory  DataStoreName=De_sum_1  ReadBeforeWriteMsg=warning  WriteAfterWriteMsg=warning  WriteAfterReadMsg=warning  ShowAdditionalParam=off  OutDataTypeStr=double  Dimensions=1
  Data Store Memory4 : DataStoreMemory  DataStoreName=De_sum_2  ReadBeforeWriteMsg=warning  WriteAfterWriteMsg=warning  WriteAfterReadMsg=warning  ShowAdditionalParam=off  OutDataTypeStr=double  Dimensions=1
  Data Store Memory5 : DataStoreMemory  DataStoreName=Send_Buffer_1  ReadBeforeWriteMsg=warning  WriteAfterWriteMsg=warning  WriteAfterReadMsg=warning  InitialValue=[101, 102, zeros(1,98)]  VectorParams1D=off  ShowAdditionalParam=off  OutDataTypeStr=double  Dimensions=[1,100]
  Data Store Memory6 : DataStoreMemory  DataStoreName=Filter  ReadBeforeWriteMsg=warning  WriteAfterWriteMsg=warning  WriteAfterReadMsg=warning  InitialValue=zeros(20,7)  VectorParams1D=off  ShowAdditionalParam=off  OutDataTypeStr=double  Dimensions=[20,7]
  Data Store Memory7 : DataStoreMemory  DataStoreName=De_1  ReadBeforeWriteMsg=warning  WriteAfterWriteMsg=warning  WriteAfterReadMsg=warning  ShowAdditionalParam=off  OutDataTypeStr=double  Dimensions=1
  Data Store Memory8 : DataStoreMemory  DataStoreName=T_send_1  ReadBeforeWriteMsg=warning  WriteAfterWriteMsg=warning  WriteAfterReadMsg=warning  ShowAdditionalParam=off  OutDataTypeStr=double  Dimensions=1
  Data Store Memory9 : DataStoreMemory  DataStoreName=T_recv_1  ReadBeforeWriteMsg=warning  WriteAfterWriteMsg=warning  WriteAfterReadMsg=warning  ShowAdditionalParam=off  OutDataTypeStr=double  Dimensions=1
  Data Store Read : DataStoreRead  DataStoreName=Send_Buffer_1
  Data Store Read1 : DataStoreRead  DataStoreName=Address
  Data Store Read10 : DataStoreRead  DataStoreName=De_sum_2
  Data Store Read11 : DataStoreRead  DataStoreName=De_sum_1
  Data Store Read12 : DataStoreRead  DataStoreName=T_send_2
  Data Store Read13 : DataStoreRead  DataStoreName=T_send_1
  Data Store Read14 : DataStoreRead  DataStoreName=T_recv_1
  Data Store Read15 : DataStoreRead  DataStoreName=T_recv_2
  Data Store Read16 : DataStoreRead  DataStoreName=De_2
  Data Store Read2 : DataStoreRead  DataStoreName=Filter
  Data Store Read3 : DataStoreRead  DataStoreName=Address_1
  Data Store Read4 : DataStoreRead  DataStoreName=Address_2
  Data Store Read5 : DataStoreRead  DataStoreName=Handshake_1
  Data Store Read6 : DataStoreRead  DataStoreName=Handshake_2
  Data Store Read7 : DataStoreRead  DataStoreName=Recv_Buffer
  Data Store Read8 : DataStoreRead  DataStoreName=Send_Buffer_2
  Data Store Read9 : DataStoreRead  DataStoreName=De_1
  Data Store Write : DataStoreWrite  DataStoreName=Address
  Delay1 : Delay  DelayLength=1
  Delay2 : Delay  DelayLength=1
  Display{,1..4,8..11,13} (10 alike) : Display
  Global_Var_Length : MATLAB Function  TreatAsAtomicUnit=on
  Memory2 : Memory  InitialCondition=false
  Recv_1 : MATLAB Function  TreatAsAtomicUnit=on  SystemSampleTime=10/f
  Recv_2 : MATLAB Function  TreatAsAtomicUnit=on  SystemSampleTime=10/f
  Send_Telegram : Subsystem
  Send_to_Host : MATLAB Function  TreatAsAtomicUnit=on  SystemSampleTime=10/f
  Status : Stateflow chart  TreatAsAtomicUnit=on
  Time : Clock
      settings: Decimation=f
  Out Bus Element : Outport  PortName=Tx_1  Element=signal
  Out Bus Element1 : Outport  PortName=Tx_1  Element=data
  Out Bus Element2 : Outport  Port=2  PortName=Tx_2  Element=signal
  Out Bus Element3 : Outport  Port=2  PortName=Tx_2  Element=data
  status : Outport  Port=3
  send_done : Outport  Port=4
  Out Bus Element4 : Outport  Port=5  PortName=Recv  Element=signal
  Out Bus Element5 : Outport  Port=5  PortName=Recv  Element=package
  wires:
  ErrorSignal/1 -> Status/1(Error_Signal)
  Status/1(status) -> [status], status/1
  In Bus Element1/1 -> Recv_1/7(Rx_1_data)
  In Bus Element/1 -> Recv_1/6(Rx_1_signal)
  [status] -> Delay1/1
  Time/1 -> [clock]
  [clock] -> Recv_1/2(clock)
  Send_to_Host/1(signal) -> Out Bus Element4/1, Memory2/1
  address/1 -> Data Store Write/1
  Global_Var_Length/1(len_Send_Buffer_1) -> [len_Send_Buffer_1]
  Global_Var_Length/2(len_Send_Buffer_2) -> [len_Send_Buffer_2]
  Global_Var_Length/3(len_Recv_Buffer) -> [len_Recv_Buffer]
  Global_Var_Length/4(len_Filter) -> [len_Filter]
  [len_Send_Buffer_1] -> Recv_1/3(lenS_1)
  [len_Send_Buffer_2] -> Recv_1/4(lenS_2)
  [len_Recv_Buffer] -> Recv_1/5(lenR)
  In Bus Element2/1 -> Recv_2/6(Rx_2_signal)
  In Bus Element3/1 -> Recv_2/7(Rx_2_data)
  [status] -> Delay2/1
  [len_Recv_Buffer] -> Recv_2/5(lenR)
  [len_Send_Buffer_1] -> Recv_2/3(lenS_1)
  [clock] -> Recv_2/2(clock)
  [len_Send_Buffer_2] -> Recv_2/4(lenS_2)
  Delay1/1 -> Recv_1/1(status)
  Delay2/1 -> Recv_2/1(status)
  Recv_1/1(recv_signal_1) -> Status/2(recv_signal_1)
  Recv_1/2(recv_package_1) -> Status/3(recv_data_1)
  Recv_2/1(recv_signal_2) -> Status/4(recv_signal_2)
  Recv_2/2(recv_package_2) -> Status/5(recv_data_2)
  [len_Recv_Buffer] -> Send_to_Host/1(lenR)
  [len_Filter] -> Send_to_Host/2(lenF)
  [len_Send_Buffer_1] -> Add_to_Send_Buffer/2(lenS_1)
  [len_Send_Buffer_2] -> Add_to_Send_Buffer/3(lenS_2)
  In Bus Element4/1 -> Add_to_Send_Buffer/4(to_send_signal)
  In Bus Element5/1 -> Add_to_Send_Buffer/5(to_send_package)
  [status] -> Add_to_Send_Buffer/1(status)
  Memory2/1 -> Send_to_Host/3(signal_old)
  Bus Creator/1 -> Display/1
  [len_Send_Buffer_1] -> Bus Creator/1
  [len_Send_Buffer_2] -> Bus Creator/2
  [len_Recv_Buffer] -> Bus Creator/3
  [len_Filter] -> Bus Creator/4
  Data Store Read/1 -> Display1/1
  Data Store Read2/1 -> Display3/1
  Data Store Read8/1 -> Display8/1
  Data Store Read7/1 -> Display9/1
  Data Store Read13/1 -> Bus Creator1/1
  Data Store Read14/1 -> Bus Creator1/2
  Data Store Read11/1 -> Bus Creator1/4
  Data Store Read9/1 -> Bus Creator1/3
  Bus Creator1/1 -> Display10/1
  Data Store Read12/1 -> Bus Creator2/1
  Data Store Read15/1 -> Bus Creator2/2
  Bus Creator2/1 -> Display11/1
  Data Store Read16/1 -> Bus Creator2/3
  Data Store Read10/1 -> Bus Creator2/4
  [status] -> Display13/1
  Send_to_Host/2(package) -> Out Bus Element5/1
  Data Store Read5/1 -> Bus Creator3/1
  Data Store Read6/1 -> Bus Creator3/2
  Data Store Read4/1 -> Bus Creator4/3
  Data Store Read1/1 -> Bus Creator4/2
  Data Store Read3/1 -> Bus Creator4/1
  Bus Creator3/1 -> Display2/1
  Bus Creator4/1 -> Display4/1
  [len_Send_Buffer_2] -> Send_Telegram/4(lenS_2)
  [clock] -> Send_Telegram/2(clock)
  [len_Send_Buffer_1] -> Send_Telegram/3(lenS_1)
  [status] -> Send_Telegram/1(status)
  Send_Telegram/1(Tx_1_signal) -> Out Bus Element/1
  Send_Telegram/2(Tx_1_data) -> Out Bus Element1/1
  Send_Telegram/3(Tx_2_signal) -> Out Bus Element2/1
  Send_Telegram/4(Tx_2_data) -> Out Bus Element3/1

== system System_Modell/Motor_1/MotionSM_1/Motor ==
  note: parameter = [delta_T, a_max, v_max, s0]
  auto_control : Inport
  parameter : Inport  Port=2
  Delay : Delay  DelayLength=1
  Display{,1..6} (7 alike) : Display
  Integrator : Integrator
  Integrator1 : Integrator
  MATLAB Function : MATLAB Function  TreatAsAtomicUnit=on
  MATLAB Function1 : MATLAB Function  TreatAsAtomicUnit=on
  MATLAB Function2 : MATLAB Function  TreatAsAtomicUnit=on
  Memory2 : Memory
  status_Motor : Outport
  a : Outport  Port=2
  v : Outport  Port=3
  s : Outport  Port=4
  wires:
  Integrator/1 -> MATLAB Function1/1(v)
  Integrator1/1 -> MATLAB Function2/1(s), Memory2/1
  auto_control/1 -> Display/1, MATLAB Function/1(Motor_control_signal)
  MATLAB Function/1(status_Motor) -> Display4/1, status_Motor/1
  parameter/1 -> Display5/1, MATLAB Function/2(parameter)
  MATLAB Function/2(a) -> a/1, Display1/1, Integrator/1  "a"
  MATLAB Function1/1(V) -> Display2/1, v/1, Delay/1, Integrator1/1  "v"
  MATLAB Function/3(direction) -> MATLAB Function1/2(direction), MATLAB Function2/3(direction), Display6/1
  MATLAB Function2/1(S) -> Display3/1, s/1  "s"
  Memory2/1 -> MATLAB Function2/2(s_old)
  Delay/1 -> MATLAB Function/3(v)

== system System_Modell/Motor_1/Schnittstelle_0/Send_Telegram ==
  status : Inport
  clock : Inport  Port=2
  lenS_1 : Inport  Port=3
  lenS_2 : Inport  Port=4
  wait2send_sgn : Inport  Port=5
  wait2send_pkg : Inport  Port=6
  Logical Operator : Logic  Operator=OR  AllPortsSameDT=off  OutDataTypeStr=boolean
  Memory : Memory  InitialCondition=false
  Memory1 : Memory  InitialCondition=false
  Pulse : DiscretePulseGenerator  PulseType=Time based  Amplitude=true  Period=200/f  PulseWidth=30
  Send_Done_1 : MATLAB Function  TreatAsAtomicUnit=on
  Send_Done_2 : MATLAB Function  TreatAsAtomicUnit=on
  Send_Telegram_1 : MATLAB Function  TreatAsAtomicUnit=on  SystemSampleTime=100/f
  Send_Telegram_2 : MATLAB Function  TreatAsAtomicUnit=on  SystemSampleTime=100/f
  Tx_1_signal : Outport
  Tx_1_data : Outport  Port=2
  Tx_2_signal : Outport  Port=3
  Tx_2_data : Outport  Port=4
  send_done : Outport  Port=5
  wires:
  status/1 -> Send_Telegram_1/1(status), Send_Telegram_2/1(status)
  clock/1 -> Send_Telegram_1/2(clock), Send_Telegram_2/2(clock)
  Send_Telegram_1/1(Tx_1_signal) -> Tx_1_signal/1, Send_Done_1/3(Tx_1_sgn), Memory/1
  lenS_1/1 -> Send_Telegram_1/3(lenS_1)
  Memory/1 -> Send_Telegram_1/5(send_1_old)
  Send_Telegram_1/2(Tx_1_data) -> Tx_1_data/1, Send_Done_1/4(Tx_1_data)
  Pulse/1 -> Send_Telegram_2/4(impulse), Send_Telegram_1/4(impulse)
  Memory1/1 -> Send_Telegram_2/5(send_2_old)
  Send_Telegram_2/1(Tx_2_signal) -> Send_Done_2/3(Tx_2_sgn), Tx_2_signal/1, Memory1/1
  Send_Telegram_2/2(Tx_2_data) -> Tx_2_data/1, Send_Done_2/4(Tx_2_data)
  lenS_2/1 -> Send_Telegram_2/3(lenS_2)
  wait2send_sgn/1 -> Send_Done_2/1(wait2send_sgn), Send_Done_1/1(wait2send_sgn)
  wait2send_pkg/1 -> Send_Done_2/2(wait2send_pkg), Send_Done_1/2(wait2send_pkg)
  Send_Done_1/1(send_done_1) -> Logical Operator/1
  Send_Done_2/1(send_done_2) -> Logical Operator/2
  Logical Operator/1 -> send_done/1

== system System_Modell/Motor_2/MotionSM_1/Motor ==
  note: parameter = [delta_T, a_max, v_max, s0]
  auto_control : Inport
  parameter : Inport  Port=2
  Delay : Delay  DelayLength=1
  Display{,1..6} (7 alike) : Display
  Integrator : Integrator
  Integrator1 : Integrator
  MATLAB Function : MATLAB Function  TreatAsAtomicUnit=on
  MATLAB Function1 : MATLAB Function  TreatAsAtomicUnit=on
  MATLAB Function2 : MATLAB Function  TreatAsAtomicUnit=on
  Memory2 : Memory
  status_Motor : Outport
  a : Outport  Port=2
  v : Outport  Port=3
  s : Outport  Port=4
  wires:
  Integrator/1 -> MATLAB Function1/1(v)
  Integrator1/1 -> MATLAB Function2/1(s), Memory2/1
  auto_control/1 -> Display/1, MATLAB Function/1(Motor_control_signal)
  MATLAB Function/1(status_Motor) -> Display4/1, status_Motor/1
  parameter/1 -> Display5/1, MATLAB Function/2(parameter)
  MATLAB Function/2(a) -> a/1, Display1/1, Integrator/1  "a"
  MATLAB Function1/1(V) -> Display2/1, v/1, Delay/1, Integrator1/1  "v"
  MATLAB Function/3(direction) -> MATLAB Function1/2(direction), MATLAB Function2/3(direction), Display6/1
  MATLAB Function2/1(S) -> Display3/1, s/1  "s"
  Memory2/1 -> MATLAB Function2/2(s_old)
  Delay/1 -> MATLAB Function/3(v)

== system System_Modell/Motor_2/Schnittstelle_0/Send_Telegram ==
  status : Inport
  clock : Inport  Port=2
  lenS_1 : Inport  Port=3
  lenS_2 : Inport  Port=4
  wait2send_sgn : Inport  Port=5
  wait2send_pkg : Inport  Port=6
  Logical Operator : Logic  Operator=OR  AllPortsSameDT=off  OutDataTypeStr=boolean
  Memory : Memory  InitialCondition=false
  Memory1 : Memory  InitialCondition=false
  Pulse : DiscretePulseGenerator  PulseType=Time based  Amplitude=true  Period=200/f  PulseWidth=30
  Send_Done_1 : MATLAB Function  TreatAsAtomicUnit=on
  Send_Done_2 : MATLAB Function  TreatAsAtomicUnit=on
  Send_Telegram_1 : MATLAB Function  TreatAsAtomicUnit=on  SystemSampleTime=100/f
  Send_Telegram_2 : MATLAB Function  TreatAsAtomicUnit=on  SystemSampleTime=100/f
  Tx_1_signal : Outport
  Tx_1_data : Outport  Port=2
  Tx_2_signal : Outport  Port=3
  Tx_2_data : Outport  Port=4
  send_done : Outport  Port=5
  wires:
  status/1 -> Send_Telegram_1/1(status), Send_Telegram_2/1(status)
  clock/1 -> Send_Telegram_1/2(clock), Send_Telegram_2/2(clock)
  Send_Telegram_1/1(Tx_1_signal) -> Tx_1_signal/1, Send_Done_1/3(Tx_1_sgn), Memory/1
  lenS_1/1 -> Send_Telegram_1/3(lenS_1)
  Memory/1 -> Send_Telegram_1/5(send_1_old)
  Send_Telegram_1/2(Tx_1_data) -> Tx_1_data/1, Send_Done_1/4(Tx_1_data)
  Pulse/1 -> Send_Telegram_2/4(impulse), Send_Telegram_1/4(impulse)
  Memory1/1 -> Send_Telegram_2/5(send_2_old)
  Send_Telegram_2/1(Tx_2_signal) -> Send_Done_2/3(Tx_2_sgn), Tx_2_signal/1, Memory1/1
  Send_Telegram_2/2(Tx_2_data) -> Tx_2_data/1, Send_Done_2/4(Tx_2_data)
  lenS_2/1 -> Send_Telegram_2/3(lenS_2)
  wait2send_sgn/1 -> Send_Done_2/1(wait2send_sgn), Send_Done_1/1(wait2send_sgn)
  wait2send_pkg/1 -> Send_Done_2/2(wait2send_pkg), Send_Done_1/2(wait2send_pkg)
  Send_Done_1/1(send_done_1) -> Logical Operator/1
  Send_Done_2/1(send_done_2) -> Logical Operator/2
  Logical Operator/1 -> send_done/1

== system System_Modell/Motor_3/MotionSM_1/Motor ==
  note: parameter = [delta_T, a_max, v_max, s0]
  auto_control : Inport
  parameter : Inport  Port=2
  Delay : Delay  DelayLength=1
  Display{,1..6} (7 alike) : Display
  Integrator : Integrator
  Integrator1 : Integrator
  MATLAB Function : MATLAB Function  TreatAsAtomicUnit=on
  MATLAB Function1 : MATLAB Function  TreatAsAtomicUnit=on
  MATLAB Function2 : MATLAB Function  TreatAsAtomicUnit=on
  Memory2 : Memory
  status_Motor : Outport
  a : Outport  Port=2
  v : Outport  Port=3
  s : Outport  Port=4
  wires:
  Integrator/1 -> MATLAB Function1/1(v)
  Integrator1/1 -> MATLAB Function2/1(s), Memory2/1
  auto_control/1 -> Display/1, MATLAB Function/1(Motor_control_signal)
  MATLAB Function/1(status_Motor) -> Display4/1, status_Motor/1
  parameter/1 -> Display5/1, MATLAB Function/2(parameter)
  MATLAB Function/2(a) -> a/1, Display1/1, Integrator/1  "a"
  MATLAB Function1/1(V) -> Display2/1, v/1, Delay/1, Integrator1/1  "v"
  MATLAB Function/3(direction) -> MATLAB Function1/2(direction), MATLAB Function2/3(direction), Display6/1
  MATLAB Function2/1(S) -> Display3/1, s/1  "s"
  Memory2/1 -> MATLAB Function2/2(s_old)
  Delay/1 -> MATLAB Function/3(v)

== system System_Modell/Motor_3/Schnittstelle_0/Send_Telegram ==
  status : Inport
  clock : Inport  Port=2
  lenS_1 : Inport  Port=3
  lenS_2 : Inport  Port=4
  wait2send_sgn : Inport  Port=5
  wait2send_pkg : Inport  Port=6
  Logical Operator : Logic  Operator=OR  AllPortsSameDT=off  OutDataTypeStr=boolean
  Memory : Memory  InitialCondition=false
  Memory1 : Memory  InitialCondition=false
  Pulse : DiscretePulseGenerator  PulseType=Time based  Amplitude=true  Period=200/f  PulseWidth=30
  Send_Done_1 : MATLAB Function  TreatAsAtomicUnit=on
  Send_Done_2 : MATLAB Function  TreatAsAtomicUnit=on
  Send_Telegram_1 : MATLAB Function  TreatAsAtomicUnit=on  SystemSampleTime=100/f
  Send_Telegram_2 : MATLAB Function  TreatAsAtomicUnit=on  SystemSampleTime=100/f
  Tx_1_signal : Outport
  Tx_1_data : Outport  Port=2
  Tx_2_signal : Outport  Port=3
  Tx_2_data : Outport  Port=4
  send_done : Outport  Port=5
  wires:
  status/1 -> Send_Telegram_1/1(status), Send_Telegram_2/1(status)
  clock/1 -> Send_Telegram_1/2(clock), Send_Telegram_2/2(clock)
  Send_Telegram_1/1(Tx_1_signal) -> Tx_1_signal/1, Send_Done_1/3(Tx_1_sgn), Memory/1
  lenS_1/1 -> Send_Telegram_1/3(lenS_1)
  Memory/1 -> Send_Telegram_1/5(send_1_old)
  Send_Telegram_1/2(Tx_1_data) -> Tx_1_data/1, Send_Done_1/4(Tx_1_data)
  Pulse/1 -> Send_Telegram_2/4(impulse), Send_Telegram_1/4(impulse)
  Memory1/1 -> Send_Telegram_2/5(send_2_old)
  Send_Telegram_2/1(Tx_2_signal) -> Send_Done_2/3(Tx_2_sgn), Tx_2_signal/1, Memory1/1
  Send_Telegram_2/2(Tx_2_data) -> Tx_2_data/1, Send_Done_2/4(Tx_2_data)
  lenS_2/1 -> Send_Telegram_2/3(lenS_2)
  wait2send_sgn/1 -> Send_Done_2/1(wait2send_sgn), Send_Done_1/1(wait2send_sgn)
  wait2send_pkg/1 -> Send_Done_2/2(wait2send_pkg), Send_Done_1/2(wait2send_pkg)
  Send_Done_1/1(send_done_1) -> Logical Operator/1
  Send_Done_2/1(send_done_2) -> Logical Operator/2
  Logical Operator/1 -> send_done/1

== system System_Modell/ZP_Mananger/GSM /ZP-Tabelle bearbeiten ==
  note: Update_data = [sender, receiver, cmd=113, n, Ax, status, delay]
  note: Skill Request: neu_ZP in der ZP-Tabelle einschreiben
  note: Status_Update: Status in der ZP-Tabelle aktualisieren
  note: 目前只能更新ZP的状态：wait, aktiv, done
      | 无法处理其他Command
  note: [7,7,111,30,40,50,1]
  status : Inport
  SkillRequest_signal : Inport  Port=2  OutDataTypeStr=boolean
  Adresse : Inport  Port=3
  SkillRequest : Inport  Port=4  OutDataTypeStr=double
  Update_signal : Inport  Port=5  OutDataTypeStr=boolean
  Update_data : Inport  Port=6  OutDataTypeStr=double
  Add : Sum
  Constant : Constant
  Constant2 : Constant  Value=2  OutDataTypeStr=double
  Display : Display
  Display3 : Display
  Logical Operator : Logic  AllPortsSameDT=off  OutDataTypeStr=boolean
  MATLAB Function : MATLAB Function  TreatAsAtomicUnit=on
  Memory : Memory
  Memory1 : Memory  InitialCondition=[0 0 0]
  Relational Operator : RelationalOperator  OutDataTypeStr=boolean  RndMeth=Simplest
  add_new_ZP : Subsystem
  send_SkillRequest : Outport
  Update_done : Outport  Port=2  OutDataTypeStr=boolean
  wires:
  Memory1/1 -> add_new_ZP/3(last_Axis)
  add_new_ZP/2(Axis_remenber) -> Memory1/1
  SkillRequest/1 -> add_new_ZP/2(SkillRequest)
  Update_signal/1 -> MATLAB Function/2(update_signal)
  Add/1 -> add_new_ZP/4(n)
  Update_data/1 -> MATLAB Function/3(update_data)  "[1x7]"
  MATLAB Function/1(ZP_update_done) -> Update_done/1
  Constant/1 -> Add/1
  SkillRequest_signal/1 -> Logical Operator/2
  Memory/1 -> Add/2
  add_new_ZP/3(n_remenber) -> Memory/1, Display3/1
  add_new_ZP/1(send_SkillRequest) -> Display/1, send_SkillRequest/1
  Relational Operator/1 -> Logical Operator/1
  Constant2/1 -> Relational Operator/2
  status/1 -> Relational Operator/1
  Logical Operator/1 -> add_new_ZP/Trigger
  Adresse/1 -> MATLAB Function/1(address), add_new_ZP/1(Adresse)
